simulink model "Lab3_number1"  (R2023b)
settings: Solver=VariableStepAuto  StartTime=0.0  StopTime=20  RelTol=1e-3
values from neighbouring files (symbols this model uses):
  G1_den = [1 0 0]    [Lab_3_number2.m]
  G1_num = [0 1]    [Lab_3_number2.m]
  G2_den = [1 1]    [Lab_3_number2.m]
  G2_num = [0 1]    [Lab_3_number2.m]
  G3_den = [1 0]    [Lab_3_number2.m]
  G3_num = [0 1]    [Lab_3_number2.m]
  G_den = [1 -2 2 -1 -2 2 1 -1 0 0 0]    [Lab_3_number1.m]    (also in Lab_3_number2.m = [4 -8 -4 14 -8 -2 2 6 4 0 0 0 0])
  G_num = [1 2]    [Lab_3_number1.m]    (also in Lab_3_number2.m = [2 -6 4 0 0 0 0 0])
  H1_den = [1 0]    [Lab_3_number2.m]
  H1_num = [0 1]    [Lab_3_number2.m]
  H2_den = [1 -1]    [Lab_3_number2.m]
  H2_num = [0 1]    [Lab_3_number2.m]
  H3_den = [1 -2]    [Lab_3_number2.m]
  H3_num = [0 1]    [Lab_3_number2.m]
settings Model: Creator=Kallistei  LastModifiedBy=Kallistei

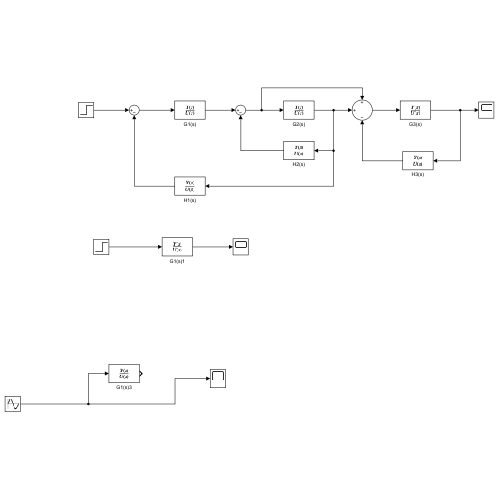
[thumbnail: Simulink's stored preview of the top-level diagram]
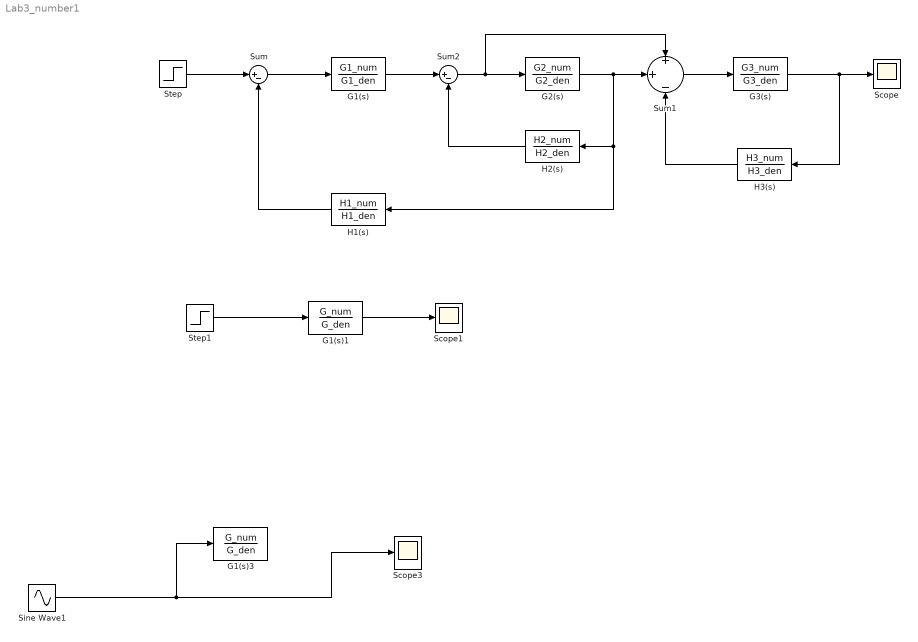
== system Lab3_number1 ==
  G1(s) : TransferFcn  Numerator=G1_num  Denominator=G1_den
  G1(s)1 : TransferFcn  Numerator=G_num  Denominator=G_den
  G1(s)3 : TransferFcn  Numerator=G_num  Denominator=G_den
  G2(s) : TransferFcn  Numerator=G2_num  Denominator=G2_den
  G3(s) : TransferFcn  Numerator=G3_num  Denominator=G3_den
  H1(s) : TransferFcn  Numerator=H1_num  Denominator=H1_den
  H2(s) : TransferFcn  Numerator=H2_num  Denominator=H2_den
  H3(s) : TransferFcn  Numerator=H3_num  Denominator=H3_den
  Scope : Scope
  Scope1 : Scope
  Scope3 : Scope
  Sine Wave1 : Sin  Amplitude=2  SampleTime=0
  Step : Step  Time=0  SampleTime=0
  Step1 : Step  Time=0  SampleTime=0
  Sum : Sum  Inputs=|+-
  Sum1 : Sum  Inputs=+||+||-
  Sum2 : Sum  Inputs=|+-
  wires:
  G3(s)/1 -> H3(s)/1, Scope/1
  Sum1/1 -> G3(s)/1
  G2(s)/1 -> H1(s)/1, H2(s)/1, Sum1/2
  H3(s)/1 -> Sum1/3
  Sum2/1 -> Sum1/1, G2(s)/1
  G1(s)/1 -> Sum2/1
  Sum/1 -> G1(s)/1
  H2(s)/1 -> Sum2/2
  H1(s)/1 -> Sum/2
  Step/1 -> Sum/1
  Step1/1 -> G1(s)1/1
  G1(s)1/1 -> Scope1/1
  Sine Wave1/1 -> G1(s)3/1, Scope3/1
